simulink model "pitch_control"  (Simulink 7.5)
settings: Solver=ode45  StartTime=0.0  StopTime=10.0  RelTol=1e-3
settings Model: Creator=Rick  LastModifiedBy=Rick

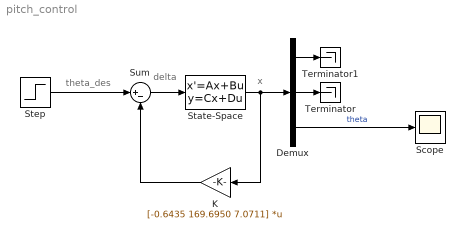
== system pitch_control ==
  note: delta
  note: theta_des
  note: x
  Demux : Demux  Outputs=3
  K : Gain  Gain=[-0.6435 169.6950 7.0711]  Multiplication=Matrix(K*u)  ParameterDataType=fixdt(1, 16)  ParameterScaling=2^0  OutDataType=fixdt(1, 16)  OutScaling=2^0
  Scope : Scope
  State-Space : StateSpace  A=[-0.313 56.7 0; -0.0139 -0.426 0; 0 56.7 0]  B=[0.232; 0.0203; 0]  C=eye(3)  D=[0;0;0]  ContinuousStateAttributes={'Angle_of_attack','Pitch_rate','Pitch_angle'}
  Step : Step  Time=0  After=0.2  SampleTime=0
  Sum : Sum  Inputs=|+-  OutDataType=fixdt(1, 16)  OutScaling=2^0
  Terminator : Terminator
  Terminator1 : Terminator
  wires:
  State-Space/1 -> K/1, Demux/1
  Step/1 -> Sum/1
  Sum/1 -> State-Space/1
  K/1 -> Sum/2
  Demux/3 -> Scope/1  "theta"
  Demux/1 -> Terminator1/1
  Demux/2 -> Terminator/1
